simulink model "cartPendulum"  (R2026a)
settings: Solver=VariableStepAuto  RelTol=1e-6
values from neighbouring files (symbols this model uses):
  c = rectangle('Parent',p)    [CartPendulum.m]    (also in setupModelParameters.m = 0.1)
  g = 9.8    [setupModelParameters.m]
  gamma = 0.005    [setupModelParameters.m]
  J = 0.006    [setupModelParameters.m]
  l = rectangle('Parent',p)    [CartPendulum.m]    (also in setupModelParameters.m = 0.3)
  M = 0.5    [setupModelParameters.m]
  m = 0.2    [setupModelParameters.m]
  xinit = [0;0.8;0;0]    [setupModelParameters.m]
settings Model: Creator=jamess  LastModifiedBy=socks

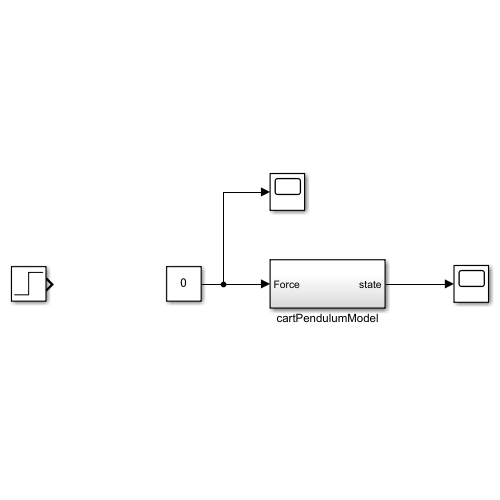
[thumbnail: Simulink's stored preview of the top-level diagram]
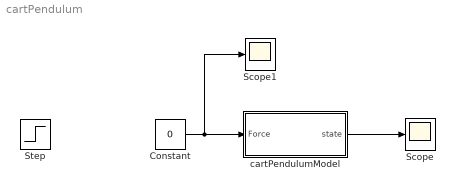
== system cartPendulum ==
  Constant : Constant  Value=0
  Scope : Scope
      settings: ActiveDisplayYMinimum=-1  ActiveDisplayYMaximum=1
  Scope1 : Scope
      settings: ActiveDisplayYMinimum=-6.25  ActiveDisplayYMaximum=6.25
  Step : Step  Time=0  FinalValue=stepFinal  SampleTime=0
  cartPendulumModel : Subsystem
  wires:
  cartPendulumModel/1(state) -> Scope/1
  Constant/1 -> Scope1/1, cartPendulumModel/1(Force)

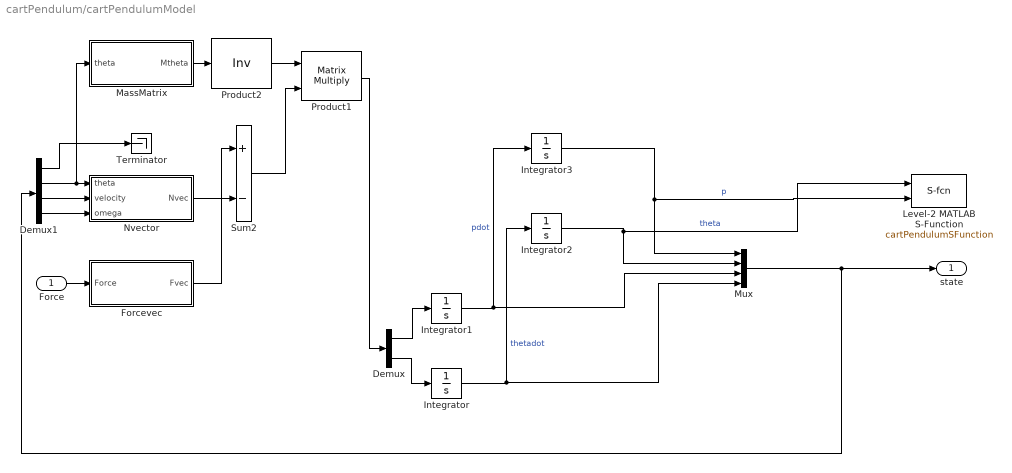
== system cartPendulum/cartPendulumModel ==
  Force : Inport
  Demux : Demux  Outputs=2
  Demux1 : Demux
  Forcevec : Subsystem
  Integrator : Integrator  InitialCondition=xinit(4)
  Integrator1 : Integrator  InitialCondition=xinit(3)
  Integrator2 : Integrator  InitialCondition=xinit(2)
  Integrator3 : Integrator  InitialCondition=xinit(1)
  Level-2 MATLAB S-Function : M-S-Function  FunctionName=cartPendulumSFunction
  MassMatrix : Subsystem
  Mux : Mux
  Nvector : Subsystem
  Product1 : Product  Multiplication=Matrix(*)
  Product2 : Product  Inputs=/  Multiplication=Matrix(*)
  Sum2 : Sum  Inputs=+-
  Terminator : Terminator
  state : Outport
  wires:
  Integrator1/1 -> Mux/3, Integrator3/1  "pdot"
  Integrator/1 -> Mux/4, Integrator2/1  "thetadot"
  Integrator3/1 -> Level-2 MATLAB S-Function/2, Mux/1  "p"
  Integrator2/1 -> Level-2 MATLAB S-Function/1, Mux/2  "theta"
  Mux/1 -> state/1, Demux1/1
  Demux/1 -> Integrator1/1
  Demux/2 -> Integrator/1
  Demux1/2 -> MassMatrix/1(theta), Nvector/1(theta)
  MassMatrix/1(Mtheta) -> Product2/1
  Product2/1 -> Product1/1
  Product1/1 -> Demux/1
  Force/1 -> Forcevec/1(Force)
  Forcevec/1(Fvec) -> Sum2/1
  Nvector/1(Nvec) -> Sum2/2
  Sum2/1 -> Product1/2
  Demux1/3 -> Nvector/2(velocity)
  Demux1/4 -> Nvector/3("omega ")
  Demux1/1 -> Terminator/1

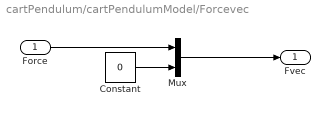
== system cartPendulum/cartPendulumModel/Forcevec ==
  Force : Inport
  Constant : Constant  Value=0
  Mux : Mux  Inputs=2
  Fvec : Outport
  wires:
  Force/1 -> Mux/1
  Mux/1 -> Fvec/1
  Constant/1 -> Mux/2

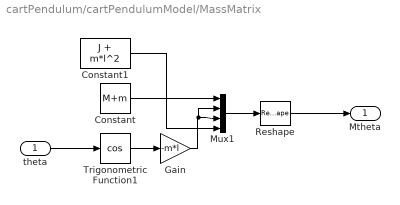
== system cartPendulum/cartPendulumModel/MassMatrix ==
  theta : Inport
  Constant : Constant  Value=M+m
  Constant1 : Constant  Value=J + m*l^2
  Gain : Gain  Gain=-m*l
  Mux1 : Mux
  Reshape : Reshape  OutputDimensionality=Customize  OutputDimensions=[2, 2]
  Trigonometric Function1 : Trigonometry  Operator=cos
  Mtheta : Outport
  wires:
  Trigonometric Function1/1 -> Gain/1
  Mux1/1 -> Reshape/1
  Constant/1 -> Mux1/1
  Gain/1 -> Mux1/3, Mux1/2
  Constant1/1 -> Mux1/4
  theta/1 -> Trigonometric Function1/1
  Reshape/1 -> Mtheta/1

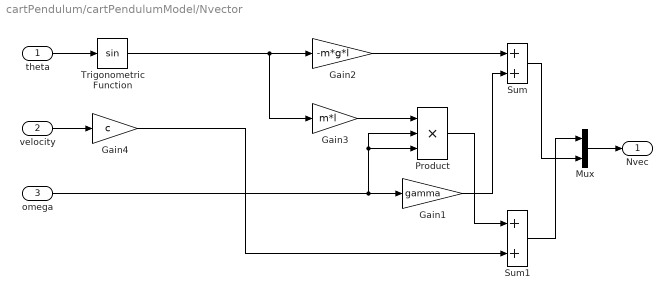
== system cartPendulum/cartPendulumModel/Nvector ==
  theta : Inport
  velocity : Inport  Port=2
  "omega " : Inport  Port=3
  Gain1 : Gain  Gain=gamma
  Gain2 : Gain  Gain=-m*g*l
  Gain3 : Gain  Gain=m*l
  Gain4 : Gain  Gain=c
  Mux : Mux  Inputs=2
  Product : Product  Inputs=3
  Sum : Sum
  Sum1 : Sum
  Trigonometric Function : Trigonometry
  Nvec : Outport
  wires:
  "omega "/1 -> Product/2, Product/3, Gain1/1
  Trigonometric Function/1 -> Gain2/1, Gain3/1
  Gain2/1 -> Sum/1
  Gain1/1 -> Sum/2
  Product/1 -> Sum1/1
  Gain3/1 -> Product/1
  Gain4/1 -> Sum1/2
  theta/1 -> Trigonometric Function/1
  velocity/1 -> Gain4/1
  Mux/1 -> Nvec/1
  Sum1/1 -> Mux/1
  Sum/1 -> Mux/2
